simulink library "Linkage_Systems"  (R2024a)
settings: Solver=VariableStepAuto  StartTime=0.0  StopTime=10.0  RelTol=1e-3
undefined symbols (not defined in the file): Init, Vehicle
libraries: Linkage_DW_B x1, Linkage_DW_Pullrod x1, Linkage_DW_Pullrod_NoSteer x1, Linkage_DW_Pushrod x1, Linkage_DW_Pushrod_NoSteer x1, Linkage_DW_A x1, Linkage_Link5C_S2LAF x1, Linkage_Link5_S2LAC_AU_NoSteer x1, Linkage_Link5_S2LAF x1, Linkage_Link5_S2LAR x1, Linkage_MacPherson x1, Linkage_MacPherson_SpLA x1
(part 1 of 2)
Description:
  | Component of Simscape Vehicle Templates Library
  | 
  | Copyright 2018-2024 The MathWorks, Inc.
settings Model: Creator=smiller  LastModifiedBy=smiller
settings SolverCC: AlgebraicLoopSolver=TrustRegion
settings DataIOCC: ReturnWorkspaceOutputs=off
settings DebuggingCC: UnconnectedInputMsg=warning  UnconnectedOutputMsg=warning  UnconnectedLineMsg=warning  ArithmeticOperatorsInVariantConditions=warning
settings ModelReferenceCC: EnableRefExpFcnMdlSchedulingChecks=on
settings SFSimCC: CustomCodeUndefinedFunction=UseInterfaceOnly
settings RTWCC: GPUComputeCapability=3.5

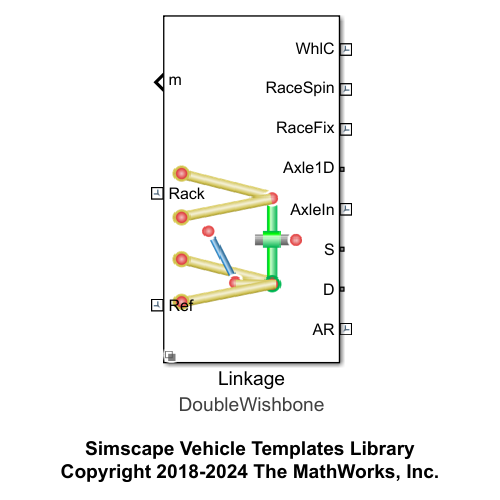
[thumbnail: Simulink's stored preview of the top-level diagram]
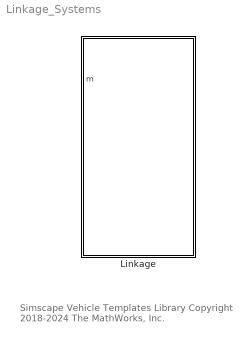
== system Linkage_Systems ==
  note: Simscape Vehicle Templates Library
      | Copyright 2018-2024 The MathWorks, Inc.
  Linkage : Subsystem  Variant=on  VariantControlMode=label  VariantControl=Variant1  LabelModeActiveChoice=DoubleWishbone  mask(Linkage){popup_leftRight=Left, Linkage=Vehicle.Chassis.SuspA1.Linkage, InitLinkage=Init.Axle1, VariantLabel=Vehicle.Chassis.SuspA1.Linkage.class.Value}
      mask prompts: popup_leftRight "Left/Right"; Linkage "Linkage Parameters"; InitLinkage "Initial Values"; VariantLabel "Variant Label"
      mask help: Select suspension linkage. Option is chosen by string provided in Variant Label. The parameters for the selected option are contained in Linkage data structure.
      mask init:
      | curblk = gcb;
      | 
      | % Set variant for this block 
      | set_param(curblk,'LabelModeActiveChoice',VariantLabel);
      | 
      | % Find other left/right blocks
      | h = sm_car_lib_find_leftright_blocks(curblk);
      | 
      | % Set left/right
      | for i=1:length(h)
      |     try % Avoid setting parameter within library links
      |         set_param(h(i),'popup_leftRight',get_param(curblk,'popup_leftRight'));
      |     end
      | end
      settings: AttributesFormatString=%<ActiveVariant>
      mask TypeOptions popup_leftRight: Left | Right
